simulink model "ThreeSpeciesSystem"  (R2024b)
settings: Solver=VariableStepAuto  StartTime=0.0  StopTime=10.0  RelTol=1e-3
undefined symbols (not defined in the file): b0, k1, k2, n, p0, s0
settings Model: Creator=JTerr  LastModifiedBy=JTerr

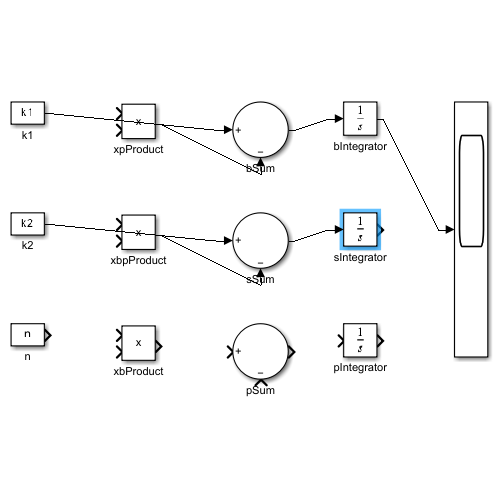
[thumbnail: Simulink's stored preview of the top-level diagram]
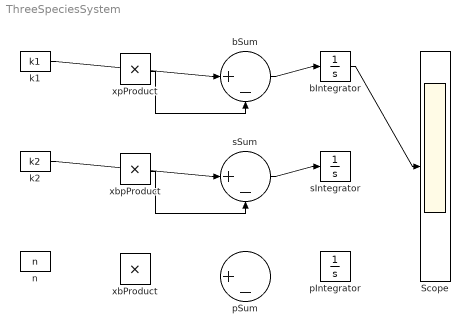
== system ThreeSpeciesSystem ==
  Scope : Scope
  bIntegrator : Integrator  InitialCondition=b0
  bSum : Sum  Inputs=|+-
  k1 : Constant  Value=k1
  k2 : Constant  Value=k2
  n : Constant  Value=n
  pIntegrator : Integrator  InitialCondition=p0
  pSum : Sum  Inputs=|+-
  sIntegrator : Integrator  InitialCondition=s0
  sSum : Sum  Inputs=|+-
  xbProduct : Product
  xbpProduct : Product
  xpProduct : Product
  wires:
  k1/1 -> bSum/1
  xpProduct/1 -> bSum/2
  bSum/1 -> bIntegrator/1
  bIntegrator/1 -> Scope/1
  k2/1 -> sSum/1
  xbpProduct/1 -> sSum/2
  sSum/1 -> sIntegrator/1
